simulink model "original_system"  (R2016a)
settings: Solver=VariableStepAuto  SolverMode=SingleTasking  StartTime=0.0  StopTime=3.5  RelTol=1e-3
undefined symbols (not defined in the file): A, B, K, X0
settings Model: Creator=卢成祥  LastModifiedBy=卢成祥
settings DataIOCC: ReturnWorkspaceOutputs=on
settings DebuggingCC: SFUnexpectedBacktrackingDiag=error  SFNoUnconditionalDefaultTransitionDiag=error
settings SFSimCC: SimUseLocalCustomCode=on
settings RTWCC: RTWUseLocalCustomCode=on
settings GRTTargetCC: TargetLangStandard=C99 (ISO)  RTWCAPISignals=on  RTWCAPIParams=on
settings ConfigComp: CovMetricSettings=dwe  CovSaveCumulativeToWorkspaceVar=off  CovSaveSingleToWorkspaceVar=off  CovExternalEMLEnable=on

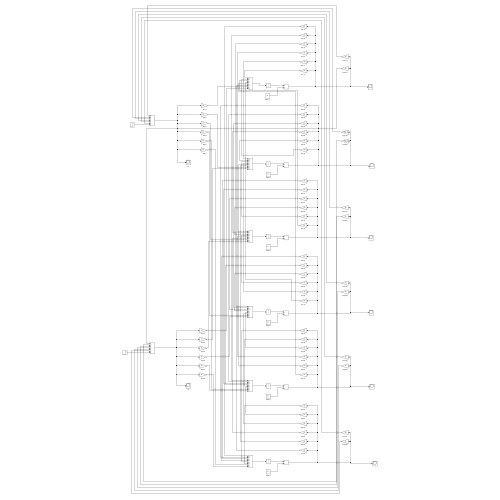
[thumbnail: Simulink's stored preview of the top-level diagram]
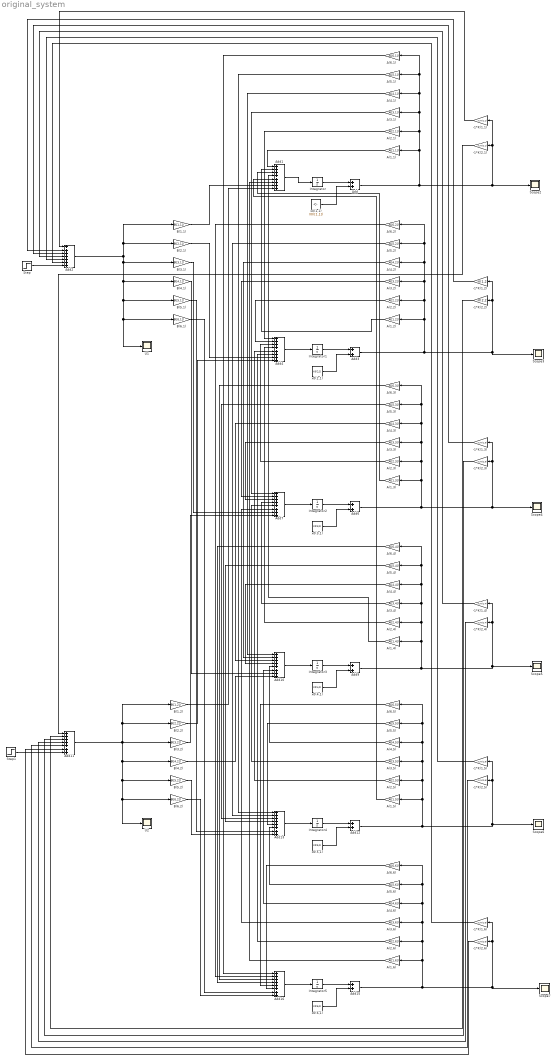
== system original_system ==
  -1*K(1,1) : Gain  Gain=-1*K(1,1)
  -1*K(1,2) : Gain  Gain=-K(1,2)
  -1*K(1,3) : Gain  Gain=-1*K(1,3)
  -1*K(1,4) : Gain  Gain=-1*K(1,4)
  -1*K(1,5) : Gain  Gain=-1*K(1,5)
  -1*K(1,6) : Gain  Gain=-1*K(1,6)
  -1*K(2,1) : Gain  Gain=-1*K(2,1)
  -1*K(2,2) : Gain  Gain=-K(2,2)
  -1*K(2,3) : Gain  Gain=-1*K(2,3)
  -1*K(2,4) : Gain  Gain=-1*K(2,4)
  -1*K(2,5) : Gain  Gain=-1*K(2,5)
  -1*K(2,6) : Gain  Gain=-1*K(2,6)
  A(1,1) : Gain  Gain=A([1,1])
  A(1,2) : Gain  Gain=A([1,2])
  A(1,3) : Gain  Gain=A([1,3])
  A(1,4) : Gain  Gain=A([1,4])
  A(1,5) : Gain  Gain=A([1,5])
  A(1,6) : Gain  Gain=A([1,6])
  A(2,1) : Gain  Gain=A([2,1])
  A(2,2) : Gain  Gain=A([2,2])
  A(2,3) : Gain  Gain=A([2,3])
  A(2,4) : Gain  Gain=A([2,4])
  A(2,5) : Gain  Gain=A([2,5])
  A(2,6) : Gain  Gain=A([2,6])
  A(3,1) : Gain  Gain=A([3,1])
  A(3,2) : Gain  Gain=A([3,2])
  A(3,3) : Gain  Gain=A([3,3])
  A(3,4) : Gain  Gain=A([3,4])
  A(3,5) : Gain  Gain=A([3,5])
  A(3,6) : Gain  Gain=A([3,6])
  A(4,1) : Gain  Gain=A([4,1])
  A(4,2) : Gain  Gain=A([4,2])
  A(4,3) : Gain  Gain=A([4,3])
  A(4,4) : Gain  Gain=A([4,4])
  A(4,5) : Gain  Gain=A([4,5])
  A(4,6) : Gain  Gain=A([4,6])
  A(5,1) : Gain  Gain=A([5,1])
  A(5,2) : Gain  Gain=A([5,2])
  A(5,3) : Gain  Gain=A([5,3])
  A(5,4) : Gain  Gain=A([5,4])
  A(5,5) : Gain  Gain=A([5,5])
  A(5,6) : Gain  Gain=A([5,6])
  A(6,1) : Gain  Gain=A([6,1])
  A(6,2) : Gain  Gain=A([6,2])
  A(6,3) : Gain  Gain=A([6,3])
  A(6,4) : Gain  Gain=A([6,4])
  A(6,5) : Gain  Gain=A([6,5])
  A(6,6) : Gain  Gain=A([6,6])
  Add{,3,6,9,12,15} (6 alike) : Sum
  Add{1,4,7,10,13,16} (6 alike) : Sum  Inputs=++++++++
  Add11 : Sum  Inputs=+++++++
  Add2 : Sum  Inputs=+++++++
  B(1,1) : Gain  Gain=B([1,1])
  B(1,2) : Gain  Gain=B([1,2])
  B(2,1) : Gain  Gain=B([2,1])
  B(2,2) : Gain  Gain=B([2,2])
  B(3,1) : Gain  Gain=B([3,1])
  B(3,2) : Gain  Gain=B([3,2])
  B(4,1) : Gain  Gain=B([4,1])
  B(4,2) : Gain  Gain=B([4,2])
  B(5,1) : Gain  Gain=B([5,1])
  B(5,2) : Gain  Gain=B([5,2])
  B(6,1) : Gain  Gain=B([6,1])
  B(6,2) : Gain  Gain=B([6,2])
  Integrator{,1..5} (6 alike) : Integrator
  Scope{2..7} (6 alike) : Scope
  Step : Step  SampleTime=0
  Step1 : Step  SampleTime=0
  U1 : Scope
  U2 : Scope
  x0(1,1) : Constant  Value=X0([1,1])
  x0(2,1) : Constant  Value=X0(2,1)
  x0(3,1) : Constant  Value=X0(3,1)
  x0(4,1) : Constant  Value=X0(4,1)
  x0(5,1) : Constant  Value=X0(5,1)
  x0(6,1) : Constant  Value=X0(6,1)
  wires:
  Integrator/1 -> Add/1
  x0(1,1)/1 -> Add/2
  Add/1 -> A(6,1)/1, A(5,1)/1, A(4,1)/1, A(3,1)/1, A(2,1)/1, A(1,1)/1, Scope2/1, -1*K(1,1)/1, -1*K(2,1)/1
  Add1/1 -> Integrator/1
  Add4/1 -> Integrator1/1
  Integrator1/1 -> Add3/1
  Add3/1 -> A(1,2)/1, A(2,2)/1, A(4,2)/1, A(5,2)/1, A(6,2)/1, A(3,2)/1, Scope3/1, -1*K(1,2)/1, -1*K(2,2)/1
  x0(2,1)/1 -> Add3/2
  Add7/1 -> Integrator2/1
  Integrator2/1 -> Add6/1
  Add6/1 -> A(2,3)/1, A(3,3)/1, A(4,3)/1, A(6,3)/1, A(5,3)/1, A(1,3)/1, Scope4/1, -1*K(1,3)/1, -1*K(2,3)/1
  x0(3,1)/1 -> Add6/2
  Add10/1 -> Integrator3/1
  Integrator3/1 -> Add9/1
  Add9/1 -> A(6,4)/1, A(5,4)/1, A(4,4)/1, A(3,4)/1, A(2,4)/1, A(1,4)/1, Scope5/1, -1*K(1,4)/1, -1*K(2,4)/1
  x0(4,1)/1 -> Add9/2
  Add13/1 -> Integrator4/1
  Integrator4/1 -> Add12/1
  Add12/1 -> A(6,5)/1, A(5,5)/1, A(4,5)/1, A(3,5)/1, A(2,5)/1, A(1,5)/1, Scope6/1, -1*K(1,5)/1, -1*K(2,5)/1
  x0(5,1)/1 -> Add12/2
  Integrator5/1 -> Add15/1
  Add15/1 -> A(2,6)/1, A(3,6)/1, A(5,6)/1, A(6,6)/1, A(4,6)/1, A(1,6)/1, Scope7/1, -1*K(1,6)/1, -1*K(2,6)/1
  x0(6,1)/1 -> Add15/2
  Add16/1 -> Integrator5/1
  A(1,1)/1 -> Add1/1
  A(1,2)/1 -> Add1/2
  A(1,3)/1 -> Add1/3
  A(1,4)/1 -> Add1/4
  A(1,5)/1 -> Add1/5
  A(1,6)/1 -> Add1/6
  B(1,1)/1 -> Add1/7
  B(1,2)/1 -> Add1/8
  B(2,1)/1 -> Add4/7
  B(2,2)/1 -> Add4/8
  A(2,1)/1 -> Add4/1
  A(2,2)/1 -> Add4/2
  A(2,3)/1 -> Add4/3
  A(2,4)/1 -> Add4/4
  A(2,5)/1 -> Add4/5
  A(2,6)/1 -> Add4/6
  A(3,1)/1 -> Add7/1
  A(3,2)/1 -> Add7/2
  A(3,3)/1 -> Add7/3
  A(3,4)/1 -> Add7/4
  A(3,5)/1 -> Add7/5
  A(3,6)/1 -> Add7/6
  B(3,1)/1 -> Add7/7
  B(3,2)/1 -> Add7/8
  A(4,1)/1 -> Add10/1
  A(4,2)/1 -> Add10/2
  A(4,3)/1 -> Add10/3
  A(4,4)/1 -> Add10/4
  A(4,5)/1 -> Add10/5
  A(4,6)/1 -> Add10/6
  B(4,2)/1 -> Add10/8
  B(4,1)/1 -> Add10/7
  B(5,2)/1 -> Add13/8
  B(6,2)/1 -> Add16/8
  B(5,1)/1 -> Add13/7
  B(6,1)/1 -> Add16/7
  A(5,1)/1 -> Add13/1
  A(5,2)/1 -> Add13/2
  A(5,3)/1 -> Add13/3
  A(5,4)/1 -> Add13/4
  A(5,5)/1 -> Add13/5
  A(5,6)/1 -> Add13/6
  A(6,1)/1 -> Add16/1
  A(6,6)/1 -> Add16/6
  A(6,5)/1 -> Add16/5
  A(6,4)/1 -> Add16/4
  A(6,3)/1 -> Add16/3
  A(6,2)/1 -> Add16/2
  -1*K(1,1)/1 -> Add2/1
  -1*K(1,2)/1 -> Add2/2
  -1*K(1,3)/1 -> Add2/3
  -1*K(1,4)/1 -> Add2/4
  -1*K(1,5)/1 -> Add2/5
  -1*K(1,6)/1 -> Add2/6
  -1*K(2,1)/1 -> Add11/1
  -1*K(2,2)/1 -> Add11/2
  -1*K(2,3)/1 -> Add11/3
  -1*K(2,4)/1 -> Add11/4
  -1*K(2,5)/1 -> Add11/5
  -1*K(2,6)/1 -> Add11/6
  Add2/1 -> U1/1, B(6,1)/1, B(5,1)/1, B(4,1)/1, B(3,1)/1, B(1,1)/1, B(2,1)/1
  Add11/1 -> U2/1, B(6,2)/1, B(5,2)/1, B(4,2)/1, B(3,2)/1, B(1,2)/1, B(2,2)/1
  Step/1 -> Add2/7
  Step1/1 -> Add11/7
